simulink model "test_snap2_10_1"  (Simulink 7.0)
settings: Solver=ode45  StartTime=0.0  StopTime=40000  RelTol=1e-3
libraries: xbsIndex_r4 x52, xps_library x7, casper_library x3
settings Model: Creator=dsp  LastModifiedBy=dsp

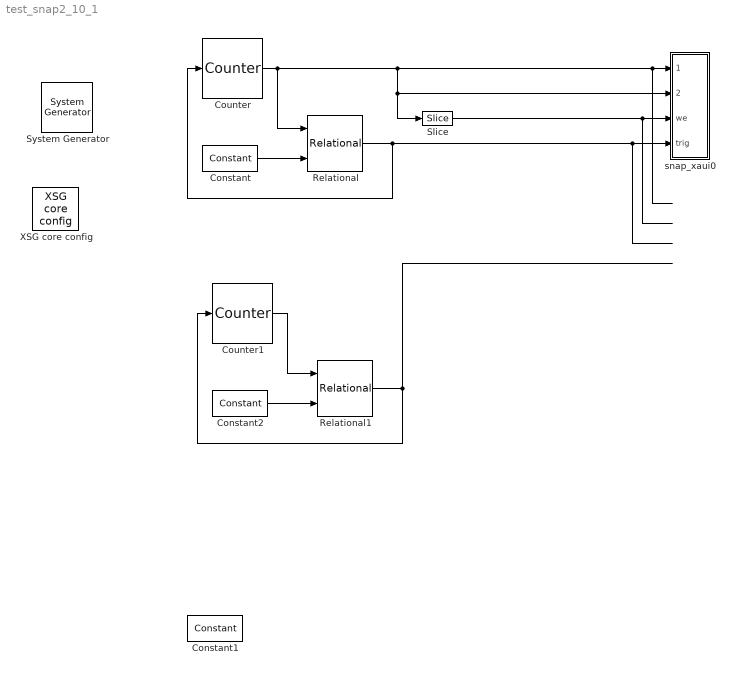
== system test_snap2_10_1 ==
  " System Generator" : xbsIndex_r4/ System Generator  Tag=genX  SystemSampleTime=-1  xilinxfamily=virtex5  part=xc5vsx95t  speed=-1  package=ff1136  synthesis_tool=XST  clock_wrapper=Clock Enables  directory=./r_4f_2x_16a_r322a/sysgen  testbench=off  simulink_period=1  sysclk_period=4.4444  dcm_input_clock_period=100  incr_netlist=off  trim_vbits=Everywhere in SubSystem  dbl_ovrd=According to Block Masks  core_generation=According to Block Masks  run_coregen=off  deprecated_control=off  eval_field=0  block_type=sysgen
      settings: block_version=10.1.3
  Constant : xbsIndex_r4/Constant  arith_type=Signed (2's comp)  const=6000  n_bits=32  bin_pt=0  explicit_period=off  period=1  equ=P=C  opselect=C  inp2=PCIN>>17  opr=+  inp1=P  carry=CIN  dbl_ovrd=off  block_type=constant
  Constant1 : xbsIndex_r4/Constant  arith_type=Boolean  const=1  n_bits=32  bin_pt=0  explicit_period=on  period=1  equ=P=C  opselect=C  inp2=PCIN>>17  opr=+  inp1=P  carry=CIN  dbl_ovrd=off  block_type=constant
  Constant2 : xbsIndex_r4/Constant  arith_type=Signed (2's comp)  const=14000  n_bits=32  bin_pt=0  explicit_period=off  period=1  equ=P=C  opselect=C  inp2=PCIN>>17  opr=+  inp1=P  carry=CIN  dbl_ovrd=off  block_type=constant
  Counter : xbsIndex_r4/Counter  cnt_type=Free Running  cnt_to=Inf  operation=Up  start_count=0  cnt_by_val=1  arith_type=Unsigned  n_bits=32  bin_pt=0  load_pin=off  rst=on  en=off  explicit_period=on  period=1  dbl_ovrd=off  use_behavioral_HDL=off  use_rpm=off  implementation=Fabric  block_type=counter
  Counter1 : xbsIndex_r4/Counter  cnt_type=Free Running  cnt_to=Inf  operation=Up  start_count=0  cnt_by_val=1  arith_type=Unsigned  n_bits=32  bin_pt=0  load_pin=off  rst=on  en=off  explicit_period=on  period=1  dbl_ovrd=off  use_behavioral_HDL=off  use_rpm=off  implementation=Fabric  block_type=counter
  Relational : xbsIndex_r4/Relational  mode=a>=b  en=off  latency=1  dbl_ovrd=off  block_type=relational
      settings: block_version=10.1.3
  Relational1 : xbsIndex_r4/Relational  mode=a>=b  en=off  latency=1  dbl_ovrd=off  block_type=relational
      settings: block_version=10.1.3
  Slice : xbsIndex_r4/Slice  nbits=1  boolean_output=on  mode=Lower Bit Location + Width  bit1=0  base1=MSB of Input  bit0=0  base0=LSB of Input  dbl_ovrd=off  block_type=slice
      settings: infoedit="Extracts a given range of bits from each input sample and presents it at the output.  The output type is ordinarily unsigned with binary point at zero, but can be Boolean when the slice is one bit wide.<P><P>Hardware notes: In hardware this block costs nothing."  block_version=10.1.3
  XSG core config : xps_library/XSG core config  Tag=xps:xsg  SystemSampleTime=-1  hw_sys=ROACH:sx95t  ibob_linux=off  clk_src=arb_clk  iBOB_clk_src=sys_clk  BEE2_ctrl_clk_src=sys_clk  BEE2_usr_clk_src=sys_clk  ROACH_clk_src=arb_clk  CORR_clk_src=sys_clk  gpio_clk_io_group=iBOB:sma  gpio_clk_bit_index=0  clk_rate=210  sample_period=1  synthesis_tool=XST  mpc_type=powerpc440_ext
  snap_xaui0 : Subsystem  mask{nsamples=12}
      mask prompts: nsamples "Number of Samples (2^?)"
  wires:
  Counter/1 -> Relational/1, Slice/1, snap_xaui0/2(oob_in), snap_xaui0/1(data_in)
  Slice/1 -> snap_xaui0/3(we)
  Relational/1 -> Counter/1, snap_xaui0/4(trig)
  Constant/1 -> Relational/2
  Counter1/1 -> Relational1/1
  Relational1/1 -> Counter1/1
  Constant2/1 -> Relational1/2

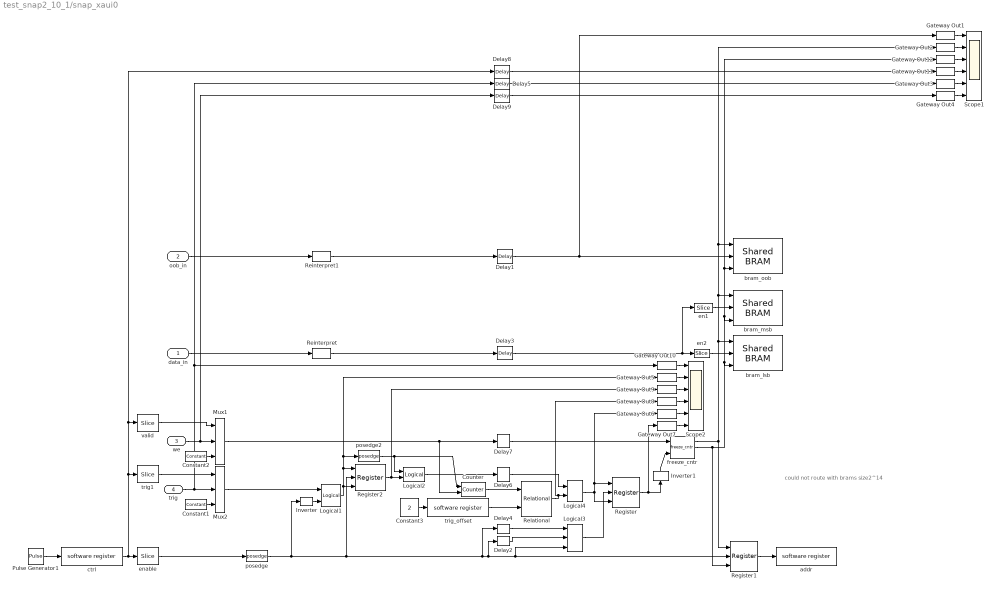
== system test_snap2_10_1/snap_xaui0 ==
  note: could not route with
      | brams size2^14
  data_in : Inport  OutDataType=sfix(16)  OutScaling=2^0
  oob_in : Inport  Port=2  OutDataType=sfix(16)  OutScaling=2^0
  we : Inport  Port=3  OutDataType=sfix(16)  OutScaling=2^0
  trig : Inport  Port=4  OutDataType=sfix(16)  OutScaling=2^0
  Constant1 : xbsIndex_r4/Constant  arith_type=Boolean  const=1  n_bits=1  bin_pt=0  explicit_period=on  period=1  equ=P=C  opselect=C  inp2=PCIN>>17  opr=+  inp1=P  carry=CIN  dbl_ovrd=off  block_type=constant
  Constant2 : xbsIndex_r4/Constant  arith_type=Boolean  const=1  n_bits=1  bin_pt=0  explicit_period=on  period=1  equ=P=C  opselect=C  inp2=PCIN>>17  opr=+  inp1=P  carry=CIN  dbl_ovrd=off  block_type=constant
  Constant3 : Constant  Value=2  OutDataType=sfix(16)  OutScaling=2^0
  Counter : xbsIndex_r4/Counter  cnt_type=Free Running  cnt_to=Inf  operation=Up  start_count=0  cnt_by_val=1  arith_type=Unsigned  n_bits=32  bin_pt=0  load_pin=off  rst=on  en=on  explicit_period=on  period=1  dbl_ovrd=off  use_behavioral_HDL=off  use_rpm=on  implementation=Fabric  block_type=counter
      settings: xl_area=[0, 0, 0, 0, 0, 0, 0]
  Delay{1,3..9} (8 alike) : xbsIndex_r4/Delay  en=off  latency=1  dbl_ovrd=off  reg_retiming=on  block_type=delay
      settings: xl_area=[0, 0, 0, 0, 0, 0, 0]
  Delay2 : xbsIndex_r4/Delay  en=off  latency=2  dbl_ovrd=off  reg_retiming=on  block_type=delay
      settings: xl_area=[0, 0, 0, 0, 0, 0, 0]
  Gateway Out{1..12} (12 alike) : xbsIndex_r4/Gateway Out  hdl_port=off  timing_constraint=None  locs_specified=off  LOCs={}  block_type=gatewayout
      settings: infoedit="Gateway out block.  Converts Xilinx fixed point inputs into ouputs of type Simulink integer, double, or fixed point.<P><P>Hardware notes:  In hardware these blocks become top level output ports or are discarded, depending on how they are configured."  xl_area=[0, 0, 0, 0, 0, 0, 0]  block_version=10.1.3
  Inverter : xbsIndex_r4/Inverter  en=off  latency=0  dbl_ovrd=off  block_type=inv
      settings: xl_area=[0, 0, 0, 0, 0, 0, 0]
  Inverter1 : xbsIndex_r4/Inverter  Orientation=up  en=off  latency=0  dbl_ovrd=off  block_type=inv
      settings: xl_area=[0, 0, 0, 0, 0, 0, 0]
  Logical1 : xbsIndex_r4/Logical  logical_function=AND  inputs=2  en=off  latency=0  precision=Full  arith_type=Unsigned  n_bits=8  bin_pt=2  align_bp=on  dbl_ovrd=off  block_type=logical
      settings: xl_area=[0, 0, 0, 0, 0, 0, 0]
  Logical2 : xbsIndex_r4/Logical  logical_function=OR  inputs=2  en=off  latency=0  precision=Full  arith_type=Unsigned  n_bits=8  bin_pt=2  align_bp=on  dbl_ovrd=off  block_type=logical
      settings: xl_area=[0, 0, 0, 0, 0, 0, 0]
  Logical3 : xbsIndex_r4/Logical  logical_function=OR  inputs=3  en=off  latency=0  precision=Full  arith_type=Unsigned  n_bits=8  bin_pt=2  align_bp=on  dbl_ovrd=off  block_type=logical
      settings: xl_area=[0, 0, 0, 0, 0, 0, 0]
  Logical4 : xbsIndex_r4/Logical  logical_function=AND  inputs=2  en=off  latency=0  precision=Full  arith_type=Unsigned  n_bits=8  bin_pt=2  align_bp=on  dbl_ovrd=off  block_type=logical
      settings: xl_area=[0, 0, 0, 0, 0, 0, 0]
  Mux1 : xbsIndex_r4/Mux  inputs=2  en=off  latency=0  precision=Full  arith_type="Signed  (2's comp)"  n_bits=8  bin_pt=2  quantization=Truncate  overflow=Wrap  dbl_ovrd=off  block_type=mux
      settings: xl_area=[0, 0, 0, 0, 0, 0, 0]
  Mux2 : xbsIndex_r4/Mux  inputs=2  en=off  latency=0  precision=Full  arith_type="Signed  (2's comp)"  n_bits=8  bin_pt=2  quantization=Truncate  overflow=Wrap  dbl_ovrd=off  block_type=mux
      settings: xl_area=[0, 0, 0, 0, 0, 0, 0]
  Pulse Generator1 : DiscretePulseGenerator  Period=25060  PulseWidth=2  PhaseDelay=100
  Register : xbsIndex_r4/Register  init=0  rst=on  en=on  dbl_ovrd=off  block_type=register
      settings: xl_area=[0, 0, 0, 0, 0, 0, 0]
  Register1 : xbsIndex_r4/Register  init=0  rst=on  en=on  dbl_ovrd=off  block_type=register
      settings: xl_area=[0, 0, 0, 0, 0, 0, 0]
  Register2 : xbsIndex_r4/Register  init=0  rst=on  en=on  dbl_ovrd=off  block_type=register
      settings: xl_area=[0, 0, 0, 0, 0, 0, 0]
  Reinterpret : xbsIndex_r4/Reinterpret  force_arith_type=on  arith_type=Unsigned  force_bin_pt=on  bin_pt=0  block_type=reinterpret
      settings: infoedit="Changes signal type without altering the binary representation.   You can changed the signal between signed and unsigned, and relocate the binary point.<P><P>Hardware notes: In hardware this block costs nothing.<P><P>Example:  Suppose the input is 6 bits wide, signed, with 2 fractional bits, and the output is forced to unsigned with 0 fractional bits.  Then an input of -2.0 (1110.00 in binary 2's complement) becomes an output of 56 (111000 in binary)."  block_version=10.1.3
  Reinterpret1 : xbsIndex_r4/Reinterpret  force_arith_type=on  arith_type=Unsigned  force_bin_pt=on  bin_pt=0  block_type=reinterpret
      settings: infoedit="Changes signal type without altering the binary representation.   You can changed the signal between signed and unsigned, and relocate the binary point.<P><P>Hardware notes: In hardware this block costs nothing.<P><P>Example:  Suppose the input is 6 bits wide, signed, with 2 fractional bits, and the output is forced to unsigned with 0 fractional bits.  Then an input of -2.0 (1110.00 in binary 2's complement) becomes an output of 56 (111000 in binary)."  block_version=10.1.3
  Relational : xbsIndex_r4/Relational  mode=a>=b  en=off  latency=0  dbl_ovrd=off  block_type=relational
      settings: xl_area=[0, 0, 0, 0, 0, 0, 0]  block_version=10.1.3
  Scope1 : Scope  NumInputPorts=6
      settings: YMin=0~0~0~0~0~0  YMax=1~1~1~1~1~1  SaveName=ScopeData2
  Scope2 : Scope  NumInputPorts=6
      settings: YMin=0~0~0~0~0~0  YMax=1~1~1~1~1~1
  addr : xps_library/software register  Tag=xps:sw_reg  SystemSampleTime=-1  io_dir=To Processor  arith_type=Unsigned  bitwidth=32  bin_pt=0  sample_period=1  gw_name=test_snap2_10_1_snap_xaui0_addr_user_data_in
      link override convert: arith_type=Unsigned  n_bits=32  bin_pt=0
  bram_lsb : xps_library/Shared BRAM  Tag=xps:bram  SystemSampleTime=-1  arith_type=Unsigned  addr_width=nsamples  data_width=32  data_bin_pt=0  init_vals=0  sample_rate=1
      link override b_2x_8a_r310b_snap_xaui0_bram_lsb_data_out: arith_type=Unsigned
      link override convert_din: arith_type=Unsigned
      link override mem/sim_data_in: arith_type=Unsigned
      link override r_2x_8a_r310b_snap_xaui0_bram_lsb_data_out: arith_type=Unsigned
      link override r_2x_8a_r311a_snap_xaui0_bram_lsb_data_out: arith_type=Unsigned
      link override r_2x_8a_r311b_1_snap_xaui0_bram_lsb_data_out: arith_type=Unsigned
      link override r_2x_8a_r311b_snap_xaui0_bram_lsb_data_out: arith_type=Unsigned
      link override r_2x_8a_r320a_1_snap_xaui0_bram_lsb_data_out: arith_type=Unsigned
      link override r_2x_8a_r320b_1_snap_xaui0_bram_lsb_data_out: arith_type=Unsigned
      link override r_2x_8a_r320b_snap_xaui0_bram_lsb_data_out: arith_type=Unsigned
      link override r_4f_2x_16a_r320b_snap_xaui0_bram_lsb_data_out: arith_type=Unsigned
      link override r_4f_2x_16a_r321a_snap_xaui0_bram_lsb_data_out: arith_type=Unsigned
      link override r_4f_2x_16a_r322a_snap_xaui0_bram_lsb_data_out: arith_type=Unsigned
      link override r_r311b_xaui_test_snap_xaui0_bram_lsb_data_out: arith_type=Unsigned
      link override test_snap2_10_1_snap_xaui0_bram_lsb_data_out: arith_type=Unsigned
  bram_msb : xps_library/Shared BRAM  Tag=xps:bram  SystemSampleTime=-1  arith_type=Unsigned  addr_width=nsamples  data_width=32  data_bin_pt=0  init_vals=0  sample_rate=1
      link override b_2x_8a_r310b_snap_xaui0_bram_msb_data_out: arith_type=Unsigned
      link override convert_din: arith_type=Unsigned
      link override mem/sim_data_in: arith_type=Unsigned
      link override r_2x_8a_r310b_snap_xaui0_bram_msb_data_out: arith_type=Unsigned
      link override r_2x_8a_r311a_snap_xaui0_bram_msb_data_out: arith_type=Unsigned
      link override r_2x_8a_r311b_1_snap_xaui0_bram_msb_data_out: arith_type=Unsigned
      link override r_2x_8a_r311b_snap_xaui0_bram_msb_data_out: arith_type=Unsigned
      link override r_2x_8a_r320a_1_snap_xaui0_bram_msb_data_out: arith_type=Unsigned
      link override r_2x_8a_r320b_1_snap_xaui0_bram_msb_data_out: arith_type=Unsigned
      link override r_2x_8a_r320b_snap_xaui0_bram_msb_data_out: arith_type=Unsigned
      link override r_4f_2x_16a_r320b_snap_xaui0_bram_msb_data_out: arith_type=Unsigned
      link override r_4f_2x_16a_r321a_snap_xaui0_bram_msb_data_out: arith_type=Unsigned
      link override r_4f_2x_16a_r322a_snap_xaui0_bram_msb_data_out: arith_type=Unsigned
      link override r_r311b_xaui_test_snap_xaui0_bram_msb_data_out: arith_type=Unsigned
      link override test_snap2_10_1_snap_xaui0_bram_msb_data_out: arith_type=Unsigned
  bram_oob : xps_library/Shared BRAM  Tag=xps:bram  SystemSampleTime=-1  arith_type=Unsigned  addr_width=nsamples  data_width=32  data_bin_pt=0  init_vals=0  sample_rate=1
      link override b_2x_8a_r310b_snap_xaui0_bram_oob_data_out: arith_type=Unsigned
      link override convert_din: arith_type=Unsigned
      link override mem/sim_data_in: arith_type=Unsigned
      link override r_2x_8a_r310b_snap_xaui0_bram_oob_data_out: arith_type=Unsigned
      link override r_2x_8a_r311a_snap_xaui0_bram_oob_data_out: arith_type=Unsigned
      link override r_2x_8a_r311b_1_snap_xaui0_bram_oob_data_out: arith_type=Unsigned
      link override r_2x_8a_r311b_snap_xaui0_bram_oob_data_out: arith_type=Unsigned
      link override r_2x_8a_r320a_1_snap_xaui0_bram_oob_data_out: arith_type=Unsigned
      link override r_2x_8a_r320b_1_snap_xaui0_bram_oob_data_out: arith_type=Unsigned
      link override r_2x_8a_r320b_snap_xaui0_bram_oob_data_out: arith_type=Unsigned
      link override r_4f_2x_16a_r320b_snap_xaui0_bram_oob_data_out: arith_type=Unsigned
      link override r_4f_2x_16a_r321a_snap_xaui0_bram_oob_data_out: arith_type=Unsigned
      link override r_4f_2x_16a_r322a_snap_xaui0_bram_oob_data_out: arith_type=Unsigned
      link override r_r311b_xaui_test_snap_xaui0_bram_oob_data_out: arith_type=Unsigned
      link override test_snap2_10_1_snap_xaui0_bram_oob_data_out: arith_type=Unsigned
  ctrl : xps_library/software register  Tag=xps:sw_reg  SystemSampleTime=-1  io_dir=From Processor  arith_type=Unsigned  bitwidth=32  bin_pt=0  sample_period=1  gw_name=test_snap2_10_1_snap_xaui0_ctrl_user_data_out
      link override b_2x_8a_r310b_snap_descramble0_ctrl_user_data_out: arith_type=Unsigned  n_bits=32  bin_pt=0  period=1
      link override r_2x_8a_r310b_snap_descramble0_ctrl_user_data_out: arith_type=Unsigned  n_bits=32  bin_pt=0  period=1
      link override r_2x_8a_r311a_snap_descramble0_ctrl_user_data_out: arith_type=Unsigned  n_bits=32  bin_pt=0  period=1
      link override r_2x_8a_r311b_1_snap_descramble0_ctrl_user_data_out: arith_type=Unsigned  n_bits=32  bin_pt=0  period=1
      link override r_2x_8a_r311b_snap_descramble0_ctrl_user_data_out: arith_type=Unsigned  n_bits=32  bin_pt=0  period=1
      link override r_2x_8a_r320a_1_snap_descramble0_ctrl_user_data_out: arith_type=Unsigned  n_bits=32  bin_pt=0  period=1
      link override r_2x_8a_r320b_1_snap_descramble0_ctrl_user_data_out: arith_type=Unsigned  n_bits=32  bin_pt=0  period=1
      link override r_2x_8a_r320b_snap_descramble0_ctrl_user_data_out: arith_type=Unsigned  n_bits=32  bin_pt=0  period=1
      link override r_4f_2x_16a_r320b_snap_descramble0_ctrl_user_data_out: arith_type=Unsigned  n_bits=32  bin_pt=0  period=1
      link override r_4f_2x_16a_r321a_snap_xaui0_ctrl_user_data_out: arith_type=Unsigned  n_bits=32  bin_pt=0  period=1
      link override r_4f_2x_16a_r322a_snap_xaui0_ctrl_user_data_out: arith_type=Unsigned  n_bits=32  bin_pt=0  period=1
      link override test_snap2_10_1_snap_xaui0_ctrl_user_data_out: arith_type=Unsigned  n_bits=32  bin_pt=0  period=1
  en1 : xbsIndex_r4/Slice  nbits=32  boolean_output=off  mode=Upper Bit Location + Width  bit1=0  base1=MSB of Input  bit0=32  base0=LSB of Input  dbl_ovrd=off  block_type=slice
      settings: infoedit="Extracts a given range of bits from each input sample and presents it at the output.  The output type is ordinarily unsigned with binary point at zero, but can be Boolean when the slice is one bit wide.<P><P>Hardware notes: In hardware this block costs nothing."  block_version=10.1.3
  en2 : xbsIndex_r4/Slice  nbits=32  boolean_output=off  mode=Lower Bit Location + Width  bit1=0  base1=LSB of Input  bit0=0  base0=LSB of Input  dbl_ovrd=off  block_type=slice
      settings: infoedit="Extracts a given range of bits from each input sample and presents it at the output.  The output type is ordinarily unsigned with binary point at zero, but can be Boolean when the slice is one bit wide.<P><P>Hardware notes: In hardware this block costs nothing."  block_version=10.1.3
  enable : xbsIndex_r4/Slice  nbits=1  boolean_output=on  mode=Lower Bit Location + Width  bit1=0  base1=LSB of Input  bit0=0  base0=LSB of Input  dbl_ovrd=off  block_type=slice
      settings: infoedit="Extracts a given range of bits from each input sample and presents it at the output.  The output type is ordinarily unsigned with binary point at zero, but can be Boolean when the slice is one bit wide.<P><P>Hardware notes: In hardware this block costs nothing."  block_version=10.1.3
  freeze_cntr : casper_library/Misc/freeze_cntr  SystemSampleTime=-1  CounterBits=nsamples
  posedge : casper_library/Misc/posedge  Tag=Rising Edge Detector  SystemSampleTime=-1
  posedge2 : casper_library/Misc/posedge  Tag=Rising Edge Detector  SystemSampleTime=-1
  trig1 : xbsIndex_r4/Slice  nbits=1  boolean_output=on  mode=Lower Bit Location + Width  bit1=0  base1=LSB of Input  bit0=1  base0=LSB of Input  dbl_ovrd=off  block_type=slice
      settings: infoedit="Extracts a given range of bits from each input sample and presents it at the output.  The output type is ordinarily unsigned with binary point at zero, but can be Boolean when the slice is one bit wide.<P><P>Hardware notes: In hardware this block costs nothing."  block_version=10.1.3
  trig_offset : xps_library/software register  Tag=xps:sw_reg  SystemSampleTime=-1  io_dir=From Processor  arith_type=Unsigned  bitwidth=32  bin_pt=0  sample_period=1  gw_name=test_snap2_10_1_snap_xaui0_trig_offset_user_data_out
      link override b_2x_8a_r310b_snap_descramble0_trig_offset_user_data_out: arith_type=Unsigned  n_bits=32  bin_pt=0  period=1
      link override r_2x_8a_r310b_snap_descramble0_trig_offset_user_data_out: arith_type=Unsigned  n_bits=32  bin_pt=0  period=1
      link override r_2x_8a_r311a_snap_descramble0_trig_offset_user_data_out: arith_type=Unsigned  n_bits=32  bin_pt=0  period=1
      link override r_2x_8a_r311b_1_snap_descramble0_trig_offset_user_data_out: arith_type=Unsigned  n_bits=32  bin_pt=0  period=1
      link override r_2x_8a_r311b_snap_descramble0_trig_offset_user_data_out: arith_type=Unsigned  n_bits=32  bin_pt=0  period=1
      link override r_2x_8a_r320a_1_snap_descramble0_trig_offset_user_data_out: arith_type=Unsigned  n_bits=32  bin_pt=0  period=1
      link override r_2x_8a_r320b_1_snap_descramble0_trig_offset_user_data_out: arith_type=Unsigned  n_bits=32  bin_pt=0  period=1
      link override r_2x_8a_r320b_snap_descramble0_trig_offset_user_data_out: arith_type=Unsigned  n_bits=32  bin_pt=0  period=1
      link override r_4f_2x_16a_r320b_snap_descramble0_trig_offset_user_data_out: arith_type=Unsigned  n_bits=32  bin_pt=0  period=1
      link override r_4f_2x_16a_r321a_snap_xaui0_trig_offset_user_data_out: arith_type=Unsigned  n_bits=32  bin_pt=0  period=1
      link override r_4f_2x_16a_r322a_snap_xaui0_trig_offset_user_data_out: arith_type=Unsigned  n_bits=32  bin_pt=0  period=1
      link override test_snap2_10_1_snap_xaui0_trig_offset_user_data_out: arith_type=Unsigned  n_bits=32  bin_pt=0  period=1
  valid : xbsIndex_r4/Slice  nbits=1  boolean_output=on  mode=Lower Bit Location + Width  bit1=0  base1=LSB of Input  bit0=2  base0=LSB of Input  dbl_ovrd=off  block_type=slice
      settings: infoedit="Extracts a given range of bits from each input sample and presents it at the output.  The output type is ordinarily unsigned with binary point at zero, but can be Boolean when the slice is one bit wide.<P><P>Hardware notes: In hardware this block costs nothing."  block_version=10.1.3
  wires:
  data_in/1 -> Reinterpret/1
  freeze_cntr/1 -> Register1/1, bram_lsb/1, bram_msb/1, bram_oob/1, Gateway Out2/1
  Register/1 -> Inverter1/1, Gateway Out7/1
  Mux2/1 -> Logical1/1
  Inverter/1 -> Logical1/2
  valid/1 -> Mux1/1
  trig1/1 -> Mux2/1
  Register1/1 -> addr/1
  Constant2/1 -> Mux1/3
  we/1 -> Mux1/2, Delay9/1
  Mux1/1 -> Counter/2, Delay7/1
  Constant1/1 -> Mux2/3
  posedge/1 -> Inverter/1, Register2/2, Delay4/1, Register1/2, Logical3/3, Delay2/1
  ctrl/1 -> trig1/1, valid/1, Delay8/1, enable/1
  freeze_cntr/2 -> Register1/3, bram_lsb/3, bram_msb/3, bram_oob/3, Gateway Out12/1
  enable/1 -> posedge/1
  trig/1 -> Mux2/2, Gateway Out10/1, Delay5/1
  Logical4/1 -> Gateway Out6/1, Register/1, Register/3
  Logical1/1 -> Register2/1, Gateway Out5/1, posedge2/1, Register2/3
  Delay3/1 -> en1/1, en2/1
  Register2/1 -> Logical2/2, Gateway Out9/1
  Delay4/1 -> Logical3/1
  Constant3/1 -> trig_offset/1
  trig_offset/1 -> Relational/2
  Relational/1 -> Logical4/2, Gateway Out8/1
  Logical2/1 -> Delay6/1
  Counter/1 -> Relational/1
  Delay2/1 -> Logical3/2
  Pulse Generator1/1 -> ctrl/1
  Reinterpret/1 -> Delay3/1
  en1/1 -> bram_msb/2
  en2/1 -> bram_lsb/2
  Delay1/1 -> bram_oob/2, Gateway Out1/1
  oob_in/1 -> Reinterpret1/1
  Reinterpret1/1 -> Delay1/1
  Gateway Out9/1 -> Scope2/3
  Gateway Out5/1 -> Scope2/2
  Gateway Out8/1 -> Scope2/4
  Gateway Out6/1 -> Scope2/5
  Gateway Out7/1 -> Scope2/6
  Gateway Out10/1 -> Scope2/1
  Inverter1/1 -> freeze_cntr/2
  Logical3/1 -> Register/2
  Delay6/1 -> Logical4/1
  Delay7/1 -> freeze_cntr/1
  Gateway Out12/1 -> Scope1/3
  Gateway Out2/1 -> Scope1/2
  Gateway Out11/1 -> Scope1/4
  Gateway Out3/1 -> Scope1/5
  Gateway Out4/1 -> Scope1/6
  Gateway Out1/1 -> Scope1/1
  Delay5/1 -> Gateway Out3/1
  Delay8/1 -> Gateway Out11/1
  Delay9/1 -> Gateway Out4/1
  posedge2/1 -> Logical2/1, Counter/1
